simulink model "Motor_COM"  (R2024a)
settings: Solver=FixedStepAuto  StartTime=0.0  StopTime=10  FixedStep=MotorSampleTime/4  RelTol=1e-3
model workspace (MAT data in the model file):
  MotorSampleTime = 0.0025
libraries: instrumentseriallib x5, sldrtlib x1
settings Model: Creator=17739  LastModifiedBy=17739

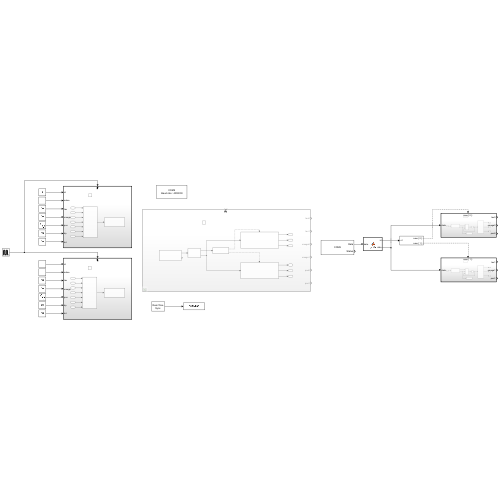
[thumbnail: Simulink's stored preview of the top-level diagram]
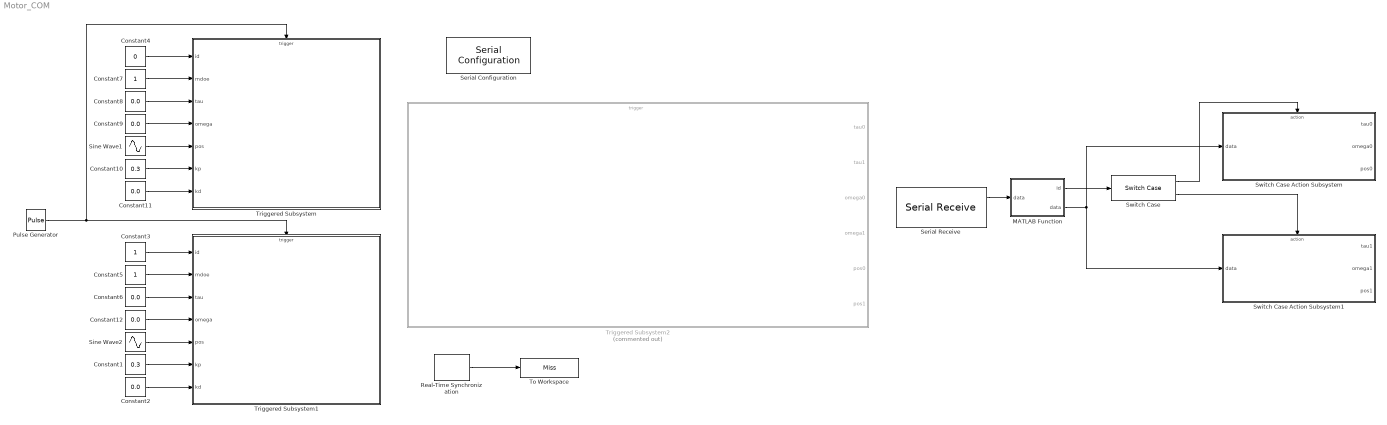
== system Motor_COM ==
  Constant1 : Constant  Value=0.3
  Constant10 : Constant  Value=0.3
  Constant{2,6,8..9,11..12} (6 alike) : Constant  Value=0.0
  Constant3 : Constant
  Constant4 : Constant  Value=0
  Constant5 : Constant
  Constant7 : Constant
  MATLAB Function : MATLAB Function  TreatAsAtomicUnit=on
  Pulse Generator : DiscretePulseGenerator  PulseType=Time based  Period=MotorSampleTime  PulseWidth=25
  Real-Time Synchronization : sldrtlib/Real-Time Synchronization  SampleTime=MotorSampleTime/4  MaxMissedTicks=inf  ShowMissedTicks=on  YieldWhenWaiting=off
  Serial Configuration : instrumentseriallib/Serial Configuration  Priority=-200000  PortSel=COM9  Port=COM9  ComPort=COM9  BaudRate=4000000  DataBits=8  Parity=none  StopBits=1  ByteOrder=little-endian  FlowControl=none  Timeout=0.02  SimulateUsing=Interpreted execution  BlockInModel=on  aMode=1
  Serial Receive : instrumentseriallib/Serial Receive  PortSel=COM9  Port=COM9  ComPort=COM9  DataType=uint8  SaveDataType=uint8  ToggleHeader=on  Header=[253 238]  ToggleDataSize=on  DataSize=14  ToggleTerminator=on  Terminator=<none>  CustomTerminator=[]  InputFormat=Row major  EnableBlockingMode=off  ActionDataUnavailable=Output last received value  ActionWhenDataUnavailable=Output last received value  CustomValue=0  SampleTime=MotorSampleTime/2  SimulateUsing=Interpreted execution  BlockInModel=on  aMode=1
  Sine Wave1 : Sin  Amplitude=pi  Frequency=pi/5  SampleTime=0
  Sine Wave2 : Sin  Amplitude=pi  Frequency=pi/5  SampleTime=0
  Switch Case : SwitchCase  CaseConditions={0,1}  ShowDefaultCase=off
  Switch Case Action Subsystem : Subsystem  TreatAsAtomicUnit=on
  Switch Case Action Subsystem1 : Subsystem  TreatAsAtomicUnit=on
  To Workspace : ToWorkspace  VariableName=Miss  SampleTime=-1
  Triggered Subsystem : Subsystem  TreatAsAtomicUnit=on
  Triggered Subsystem1 : Subsystem  TreatAsAtomicUnit=on
  Triggered Subsystem2 : Subsystem  Commented=on  TreatAsAtomicUnit=on
  wires:
  Real-Time Synchronization/1 -> To Workspace/1
  Switch Case/1 -> Switch Case Action Subsystem/Action
  Switch Case/2 -> Switch Case Action Subsystem1/Action
  MATLAB Function/2(data) -> Switch Case Action Subsystem1/1(data), Switch Case Action Subsystem/1(data)
  MATLAB Function/1(id) -> Switch Case/1
  Serial Receive/1 -> MATLAB Function/1("data ")
  Constant8/1 -> Triggered Subsystem/3(tau)
  Constant1/1 -> Triggered Subsystem1/6(kp)
  Constant6/1 -> Triggered Subsystem1/3(tau)
  Constant5/1 -> Triggered Subsystem1/2(mdoe)
  Constant9/1 -> Triggered Subsystem/4(omega)
  Constant10/1 -> Triggered Subsystem/6(kp)
  Constant4/1 -> Triggered Subsystem/1(id)
  Constant12/1 -> Triggered Subsystem1/4(omega)
  Pulse Generator/1 -> Triggered Subsystem/Trigger, Triggered Subsystem1/Trigger
  Constant11/1 -> Triggered Subsystem/7(kd)
  Constant3/1 -> Triggered Subsystem1/1(id)
  Constant2/1 -> Triggered Subsystem1/7(kd)
  Constant7/1 -> Triggered Subsystem/2(mdoe)
  Sine Wave2/1 -> Triggered Subsystem1/5(pos)
  Sine Wave1/1 -> Triggered Subsystem/5(pos)

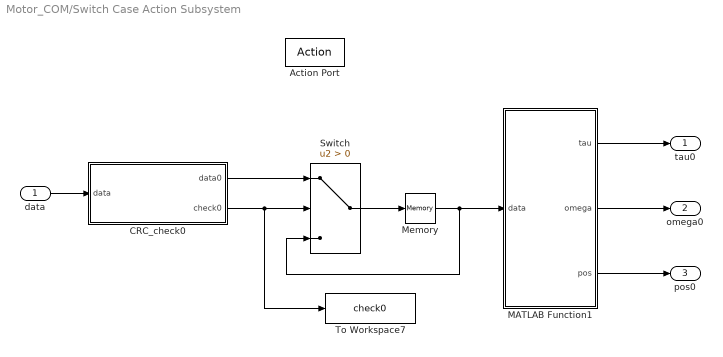
== system Motor_COM/Switch Case Action Subsystem ==
  data : Inport
  Action Port : ActionPort  ActionPortLabel=case [ 0 ]:
  CRC_check0 : MATLAB Function  TreatAsAtomicUnit=on
  MATLAB Function1 : MATLAB Function  TreatAsAtomicUnit=on
  Memory : Memory  InheritSampleTime=on
  Switch : Switch  Criteria=u2 > Threshold  SaturateOnIntegerOverflow=off  InputSameDT=off
  To Workspace7 : ToWorkspace  VariableName=check0  SampleTime=-1
  tau0 : Outport
  omega0 : Outport  Port=2
  pos0 : Outport  Port=3
  wires:
  CRC_check0/1(data0) -> Switch/1
  CRC_check0/2(check0) -> Switch/2, To Workspace7/1
  Memory/1 -> MATLAB Function1/1(data), Switch/3
  Switch/1 -> Memory/1
  data/1 -> CRC_check0/1(data)
  MATLAB Function1/1(tau) -> tau0/1
  MATLAB Function1/2(omega) -> omega0/1
  MATLAB Function1/3(pos) -> pos0/1

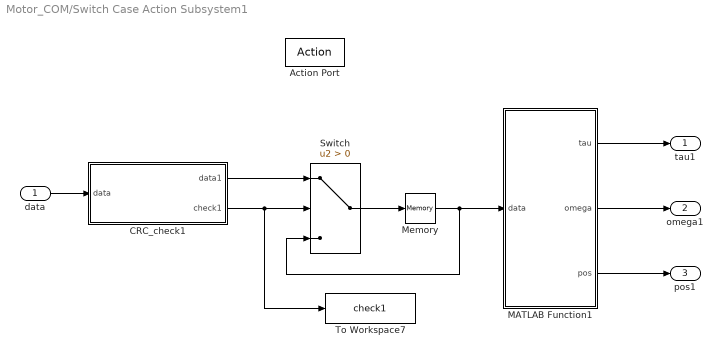
== system Motor_COM/Switch Case Action Subsystem1 ==
  data : Inport
  Action Port : ActionPort  ActionPortLabel=case [ 1 ]:
  CRC_check1 : MATLAB Function  TreatAsAtomicUnit=on
  MATLAB Function1 : MATLAB Function  TreatAsAtomicUnit=on
  Memory : Memory  InheritSampleTime=on
  Switch : Switch  Criteria=u2 > Threshold  SaturateOnIntegerOverflow=off  InputSameDT=off
  To Workspace7 : ToWorkspace  VariableName=check1  SampleTime=-1
  tau1 : Outport
  omega1 : Outport  Port=2
  pos1 : Outport  Port=3
  wires:
  CRC_check1/1(data1) -> Switch/1
  CRC_check1/2(check1) -> Switch/2, To Workspace7/1
  Memory/1 -> MATLAB Function1/1(data), Switch/3
  Switch/1 -> Memory/1
  data/1 -> CRC_check1/1(data)
  MATLAB Function1/1(tau) -> tau1/1
  MATLAB Function1/2(omega) -> omega1/1
  MATLAB Function1/3(pos) -> pos1/1

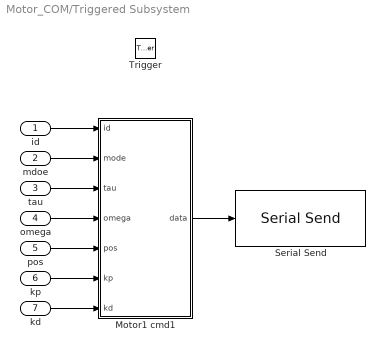
== system Motor_COM/Triggered Subsystem ==
  id : Inport
  mdoe : Inport  Port=2
  tau : Inport  Port=3
  omega : Inport  Port=4
  pos : Inport  Port=5
  kp : Inport  Port=6
  kd : Inport  Port=7
  Trigger : TriggerPort  VariantControl=(inherit)
  Motor1 cmd1 : MATLAB Function  TreatAsAtomicUnit=on
  Serial Send : instrumentseriallib/Serial Send  Priority=1  PortSel=COM9  Port=COM9  ComPort=COM9  Header=[]  Terminator=<none>  CustomTerminator=[]  EnableBlockingMode=off  SimulateUsing=Interpreted execution  BlockInModel=on  aMode=1
      settings: LibrarySourceBlock=c2000lib/Host Communication/Serial Send
  wires:
  tau/1 -> Motor1 cmd1/3(tau)
  mdoe/1 -> Motor1 cmd1/2(mode)
  kp/1 -> Motor1 cmd1/6(kp)
  id/1 -> Motor1 cmd1/1(id)
  omega/1 -> Motor1 cmd1/4(omega)
  kd/1 -> Motor1 cmd1/7(kd)
  pos/1 -> Motor1 cmd1/5(pos)
  Motor1 cmd1/1(data) -> Serial Send/1

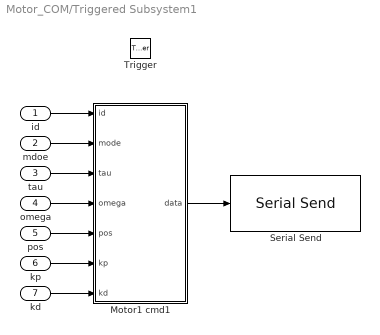
== system Motor_COM/Triggered Subsystem1 ==
  id : Inport
  mdoe : Inport  Port=2
  tau : Inport  Port=3
  omega : Inport  Port=4
  pos : Inport  Port=5
  kp : Inport  Port=6
  kd : Inport  Port=7
  Trigger : TriggerPort  TriggerType=falling  VariantControl=(inherit)
  Motor1 cmd1 : MATLAB Function  TreatAsAtomicUnit=on
  Serial Send : instrumentseriallib/Serial Send  Priority=1  PortSel=COM9  Port=COM9  ComPort=COM9  Header=[]  Terminator=<none>  CustomTerminator=[]  EnableBlockingMode=off  SimulateUsing=Interpreted execution  BlockInModel=on  aMode=1
      settings: LibrarySourceBlock=c2000lib/Host Communication/Serial Send
  wires:
  tau/1 -> Motor1 cmd1/3(tau)
  mdoe/1 -> Motor1 cmd1/2(mode)
  kp/1 -> Motor1 cmd1/6(kp)
  id/1 -> Motor1 cmd1/1(id)
  omega/1 -> Motor1 cmd1/4(omega)
  kd/1 -> Motor1 cmd1/7(kd)
  pos/1 -> Motor1 cmd1/5(pos)
  Motor1 cmd1/1(data) -> Serial Send/1

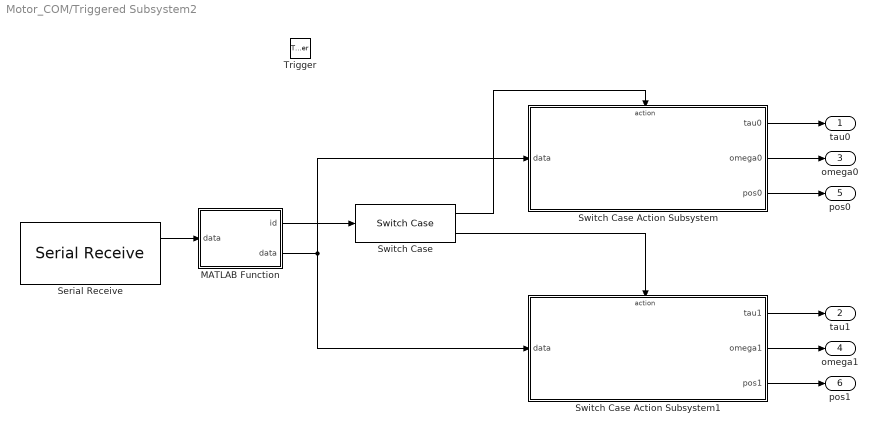
== system Motor_COM/Triggered Subsystem2 ==
  Trigger : TriggerPort  TriggerType=either  VariantControl=(inherit)
  MATLAB Function : MATLAB Function  TreatAsAtomicUnit=on
  Serial Receive : instrumentseriallib/Serial Receive  PortSel=COM9  Port=COM9  ComPort=COM9  DataType=uint8  SaveDataType=uint8  ToggleHeader=on  Header=[253 238]  ToggleDataSize=on  DataSize=14  ToggleTerminator=off  Terminator=<none>  CustomTerminator=[]  InputFormat=Row major  EnableBlockingMode=off  ActionDataUnavailable=Output last received value  ActionWhenDataUnavailable=Output last received value  CustomValue=0  SampleTime=-1  SimulateUsing=Interpreted execution  BlockInModel=on  aMode=1
  Switch Case : SwitchCase  CaseConditions={0,1}  ShowDefaultCase=off
  Switch Case Action Subsystem : Subsystem  TreatAsAtomicUnit=on
  Switch Case Action Subsystem1 : Subsystem  TreatAsAtomicUnit=on
  tau0 : Outport
  tau1 : Outport  Port=2
  omega0 : Outport  Port=3
  omega1 : Outport  Port=4
  pos0 : Outport  Port=5
  pos1 : Outport  Port=6
  wires:
  Serial Receive/1 -> MATLAB Function/1("data ")
  MATLAB Function/1(id) -> Switch Case/1
  MATLAB Function/2(data) -> Switch Case Action Subsystem1/1(data), Switch Case Action Subsystem/1(data)
  Switch Case/1 -> Switch Case Action Subsystem/Action
  Switch Case/2 -> Switch Case Action Subsystem1/Action
  Switch Case Action Subsystem/1(tau0) -> tau0/1
  Switch Case Action Subsystem1/1(tau1) -> tau1/1
  Switch Case Action Subsystem/2(omega0) -> omega0/1
  Switch Case Action Subsystem1/2(omega1) -> omega1/1
  Switch Case Action Subsystem/3(pos0) -> pos0/1
  Switch Case Action Subsystem1/3(pos1) -> pos1/1

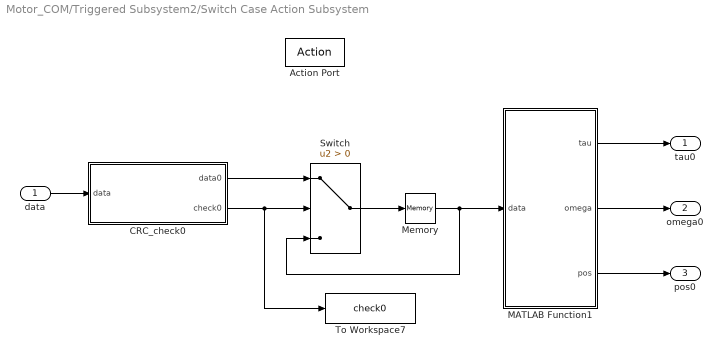
== system Motor_COM/Triggered Subsystem2/Switch Case Action Subsystem ==
  data : Inport
  Action Port : ActionPort  ActionPortLabel=case [ 0 ]:
  CRC_check0 : MATLAB Function  TreatAsAtomicUnit=on
  MATLAB Function1 : MATLAB Function  TreatAsAtomicUnit=on
  Memory : Memory  InheritSampleTime=on
  Switch : Switch  Criteria=u2 > Threshold  SaturateOnIntegerOverflow=off  InputSameDT=off
  To Workspace7 : ToWorkspace  VariableName=check0  SampleTime=-1
  tau0 : Outport
  omega0 : Outport  Port=2
  pos0 : Outport  Port=3
  wires:
  CRC_check0/1(data0) -> Switch/1
  CRC_check0/2(check0) -> Switch/2, To Workspace7/1
  Memory/1 -> MATLAB Function1/1(data), Switch/3
  Switch/1 -> Memory/1
  data/1 -> CRC_check0/1(data)
  MATLAB Function1/1(tau) -> tau0/1
  MATLAB Function1/2(omega) -> omega0/1
  MATLAB Function1/3(pos) -> pos0/1

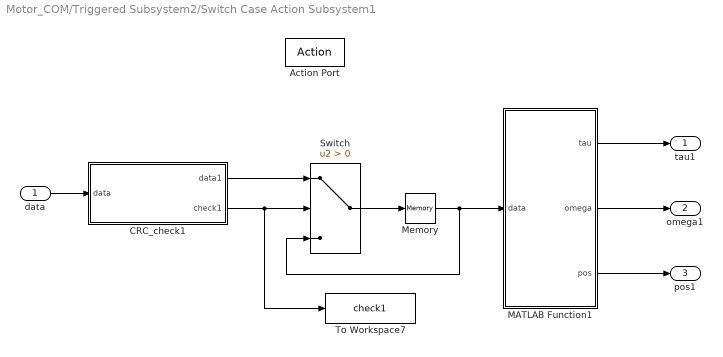
== system Motor_COM/Triggered Subsystem2/Switch Case Action Subsystem1 ==
  data : Inport
  Action Port : ActionPort  ActionPortLabel=case [ 1 ]:
  CRC_check1 : MATLAB Function  TreatAsAtomicUnit=on
  MATLAB Function1 : MATLAB Function  TreatAsAtomicUnit=on
  Memory : Memory  InheritSampleTime=on
  Switch : Switch  Criteria=u2 > Threshold  SaturateOnIntegerOverflow=off  InputSameDT=off
  To Workspace7 : ToWorkspace  VariableName=check1  SampleTime=-1
  tau1 : Outport
  omega1 : Outport  Port=2
  pos1 : Outport  Port=3
  wires:
  CRC_check1/1(data1) -> Switch/1
  CRC_check1/2(check1) -> Switch/2, To Workspace7/1
  Memory/1 -> MATLAB Function1/1(data), Switch/3
  Switch/1 -> Memory/1
  data/1 -> CRC_check1/1(data)
  MATLAB Function1/1(tau) -> tau1/1
  MATLAB Function1/2(omega) -> omega1/1
  MATLAB Function1/3(pos) -> pos1/1

== matlab function Motor_COM/Triggered Subsystem2/Switch Case Action Subsystem1/CRC_check1 ==
  data: data1 output; check1 output; data input
function [data1, check1] = CRC_Check1(data)
crc_ccitt_table = [
    0x0000, 0x1189, 0x2312, 0x329b, 0x4624, 0x57ad, 0x6536, 0x74bf, ...
    0x8c48, 0x9dc1, 0xaf5a, 0xbed3, 0xca6c, 0xdbe5, 0xe97e, 0xf8f7, ...
    0x1081, 0x0108, 0x3393, 0x221a, 0x56a5, 0x472c, 0x75b7, 0x643e, ...
    0x9cc9, 0x8d40, 0xbfdb, 0xae52, 0xdaed, 0xcb64, 0xf9ff, 0xe876, ...
    0x2102, 0x308b, 0x0210, 0x1399, 0x6726, 0x76af, 0x4434, 0x55bd, ...
    0xad4a, 0xbcc3, 0x8e58, 0x9fd1, 0xeb6e, 0xfae7, 0xc87c, 0xd9f5, ...
    0x3183, 0x200a, 0x1291, 0x0318, 0x77a7, 0x662e, 0x54b5, 0x453c, ...
    0xbdcb, 0xac42, 0x9ed9, 0x8f50, 0xfbef, 0xea66, 0xd8fd, 0xc974, ...
    0x4204, 0x538d, 0x6116, 0x709f, 0x0420, 0x15a9, 0x2732, 0x36bb, ...
    0xce4c, 0xdfc5, 0xed5e, 0xfcd7, 0x8868, 0x99e1, 0xab7a, 0xbaf3, ...
    0x5285, 0x430c, 0x7197, 0x601e, 0x14a1, 0x0528, 0x37b3, 0x263a, ...
    0xdecd, 0xcf44, 0xfddf, 0xec56, 0x98e9, 0x8960, 0xbbfb, 0xaa72, ...
    0x6306, 0x728f, 0x4014, 0x519d, 0x2522, 0x34ab, 0x0630, 0x17b9, ...
    0xef4e, 0xfec7, 0xcc5c, 0xddd5, 0xa96a, 0xb8e3, 0x8a78, 0x9bf1, ...
    0x7387, 0x620e, 0x5095, 0x411c, 0x35a3, 0x242a, 0x16b1, 0x0738, ...
    0xffcf, 0xee46, 0xdcdd, 0xcd54, 0xb9eb, 0xa862, 0x9af9, 0x8b70, ...
    0x8408, 0x9581, 0xa71a, 0xb693, 0xc22c, 0xd3a5, 0xe13e, 0xf0b7, ...
    0x0840, 0x19c9, 0x2b52, 0x3adb, 0x4e64, 0x5fed, 0x6d76, 0x7cff, ...
    0x9489, 0x8500, 0xb79b, 0xa612, 0xd2ad, 0xc324, 0xf1bf, 0xe036, ...
    0x18c1, 0x0948, 0x3bd3, 0x2a5a, 0x5ee5, 0x4f6c, 0x7df7, 0x6c7e, ...
    0xa50a, 0xb483, 0x8618, 0x9791, 0xe32e, 0xf2a7, 0xc03c, 0xd1b5, ...
    0x2942, 0x38cb, 0x0a50, 0x1bd9, 0x6f66, 0x7eef, 0x4c74, 0x5dfd, ...
    0xb58b, 0xa402, 0x9699, 0x8710, 0xf3af, 0xe226, 0xd0bd, 0xc134, ...
    0x39c3, 0x284a, 0x1ad1, 0x0b58, 0x7fe7, 0x6e6e, 0x5cf5, 0x4d7c, ...
    0xc60c, 0xd785, 0xe51e, 0xf497, 0x8028, 0x91a1, 0xa33a, 0xb2b3, ...
    0x4a44, 0x5bcd, 0x6956, 0x78df, 0x0c60, 0x1de9, 0x2f72, 0x3efb, ...
    0xd68d, 0xc704, 0xf59f, 0xe416, 0x90a9, 0x8120, 0xb3bb, 0xa232, ...
    0x5ac5, 0x4b4c, 0x79d7, 0x685e, 0x1ce1, 0x0d68, 0x3ff3, 0x2e7a, ...
    0xe70e, 0xf687, 0xc41c, 0xd595, 0xa12a, 0xb0a3, 0x8238, 0x93b1, ...
    0x6b46, 0x7acf, 0x4854, 0x59dd, 0x2d62, 0x3ceb, 0x0e70, 0x1ff9, ...
    0xf78f, 0xe606, 0xd49d, 0xc514, 0xb1ab, 0xa022, 0x92b9, 0x8330, ...
    0x7bc7, 0x6a4e, 0x58d5, 0x495c, 0x3de3, 0x2c6a, 0x1ef1, 0x0f78 ...
    ];

data1 = [253; 238; data];
crc = uint16(0);
for i = 1:14
    tableIndex = bitand(bitxor(crc, uint16(data1(i))), uint16(0xff));
    crc = bitxor(bitshift(crc, -8), crc_ccitt_table(tableIndex + 1));
end
check1 = false;
if typecast(uint8(data1(end-1:end)), 'uint16') == crc
    check1 = true;
end
end

== matlab function Motor_COM/Triggered Subsystem2/Switch Case Action Subsystem1/MATLAB Function1 ==
  data: data input size=[16 1]; tau output size=1; omega output size=1; pos output size=1
function [tau, omega, pos] = MotorData(data)
tau = double(typecast(uint8(data(4:5)), 'int16')) / 256;
omega = double(typecast(uint8(data(6:7)), 'int16')) / 256 * 2 * pi;
pos = double(typecast(uint8(data(8:11)), 'int32')) / 32768 * 2 * pi;
end

== matlab function Motor_COM/Triggered Subsystem/Motor1 cmd1 ==
  data: data output size=[1 17]; id input; mode input; tau input; omega input; pos input; kp input; kd input
function data = MotorCmd(id, mode, tau, omega, pos, kp, kd)
data = uint8([hex2dec('FE'), hex2dec('EE'), ...
    mode*16 + id, ...
    typecast(int16(fix(tau * 256)), 'uint8'), ...
    typecast(int16(fix(omega / (2 * pi) * 256)), 'uint8'), ...
    typecast(int32(fix(pos / (2 * pi) * 32768)), 'uint8'), ...
    typecast(int16(fix(kp * 1280)), 'uint8'), ...
    typecast(int16(fix(kd * 1280)), 'uint8'), ...
    0, 0]); % CRC16 计算稍后添加

% 计算并添加 CRC16 校验
crc = calculateCRC(data(1:end-2)); % 自定义 CRC 计算函数
data(end-1:end) = typecast(uint16(crc), 'uint8');
end

% 自定义 CRC 计算函数
function crc = calculateCRC(data)
crc_ccitt_table = [
    0x0000, 0x1189, 0x2312, 0x329b, 0x4624, 0x57ad, 0x6536, 0x74bf, ...
    0x8c48, 0x9dc1, 0xaf5a, 0xbed3, 0xca6c, 0xdbe5, 0xe97e, 0xf8f7, ...
    0x1081, 0x0108, 0x3393, 0x221a, 0x56a5, 0x472c, 0x75b7, 0x643e, ...
    0x9cc9, 0x8d40, 0xbfdb, 0xae52, 0xdaed, 0xcb64, 0xf9ff, 0xe876, ...
    0x2102, 0x308b, 0x0210, 0x1399, 0x6726, 0x76af, 0x4434, 0x55bd, ...
    0xad4a, 0xbcc3, 0x8e58, 0x9fd1, 0xeb6e, 0xfae7, 0xc87c, 0xd9f5, ...
    0x3183, 0x200a, 0x1291, 0x0318, 0x77a7, 0x662e, 0x54b5, 0x453c, ...
    0xbdcb, 0xac42, 0x9ed9, 0x8f50, 0xfbef, 0xea66, 0xd8fd, 0xc974, ...
    0x4204, 0x538d, 0x6116, 0x709f, 0x0420, 0x15a9, 0x2732, 0x36bb, ...
    0xce4c, 0xdfc5, 0xed5e, 0xfcd7, 0x8868, 0x99e1, 0xab7a, 0xbaf3, ...
    0x5285, 0x430c, 0x7197, 0x601e, 0x14a1, 0x0528, 0x37b3, 0x263a, ...
    0xdecd, 0xcf44, 0xfddf, 0xec56, 0x98e9, 0x8960, 0xbbfb, 0xaa72, ...
    0x6306, 0x728f, 0x4014, 0x519d, 0x2522, 0x34ab, 0x0630, 0x17b9, ...
    0xef4e, 0xfec7, 0xcc5c, 0xddd5, 0xa96a, 0xb8e3, 0x8a78, 0x9bf1, ...
    0x7387, 0x620e, 0x5095, 0x411c, 0x35a3, 0x242a, 0x16b1, 0x0738, ...
    0xffcf, 0xee46, 0xdcdd, 0xcd54, 0xb9eb, 0xa862, 0x9af9, 0x8b70, ...
    0x8408, 0x9581, 0xa71a, 0xb693, 0xc22c, 0xd3a5, 0xe13e, 0xf0b7, ...
    0x0840, 0x19c9, 0x2b52, 0x3adb, 0x4e64, 0x5fed, 0x6d76, 0x7cff, ...
    0x9489, 0x8500, 0xb79b, 0xa612, 0xd2ad, 0xc324, 0xf1bf, 0xe036, ...
    0x18c1, 0x0948, 0x3bd3, 0x2a5a, 0x5ee5, 0x4f6c, 0x7df7, 0x6c7e, ...
    0xa50a, 0xb483, 0x8618, 0x9791, 0xe32e, 0xf2a7, 0xc03c, 0xd1b5, ...
    0x2942, 0x38cb, 0x0a50, 0x1bd9, 0x6f66, 0x7eef, 0x4c74, 0x5dfd, ...
    0xb58b, 0xa402, 0x9699, 0x8710, 0xf3af, 0xe226, 0xd0bd, 0xc134, ...
    0x39c3, 0x284a, 0x1ad1, 0x0b58, 0x7fe7, 0x6e6e, 0x5cf5, 0x4d7c, ...
    0xc60c, 0xd785, 0xe51e, 0xf497, 0x8028, 0x91a1, 0xa33a, 0xb2b3, ...
    0x4a44, 0x5bcd, 0x6956, 0x78df, 0x0c60, 0x1de9, 0x2f72, 0x3efb, ...
    0xd68d, 0xc704, 0xf59f, 0xe416, 0x90a9, 0x8120, 0xb3bb, 0xa232, ...
    0x5ac5, 0x4b4c, 0x79d7, 0x685e, 0x1ce1, 0x0d68, 0x3ff3, 0x2e7a, ...
    0xe70e, 0xf687, 0xc41c, 0xd595, 0xa12a, 0xb0a3, 0x8238, 0x93b1, ...
    0x6b46, 0x7acf, 0x4854, 0x59dd, 0x2d62, 0x3ceb, 0x0e70, 0x1ff9, ...
    0xf78f, 0xe606, 0xd49d, 0xc514, 0xb1ab, 0xa022, 0x92b9, 0x8330, ...
    0x7bc7, 0x6a4e, 0x58d5, 0x495c, 0x3de3, 0x2c6a, 0x1ef1, 0x0f78 ...
    ];

crc = uint16(0);
for i = 1:length(data)
    tableIndex = bitand(bitxor(crc, uint16(data(i))), uint16(0xff));
    crc = bitxor(bitshift(crc, -8), crc_ccitt_table(tableIndex + 1));
end
end

== matlab function Motor_COM/MATLAB Function ==
  data: data input; id output; data output
function [id, data] = getID(data)
id = uint8(data(1)) - 16;
end

== matlab function Motor_COM/Triggered Subsystem1/Motor1 cmd1 ==
  data: data output size=[1 17]; id input; mode input; tau input; omega input; pos input; kp input; kd input
function data = MotorCmd(id, mode, tau, omega, pos, kp, kd)
data = uint8([hex2dec('FE'), hex2dec('EE'), ...
    mode*16 + id, ...
    typecast(int16(fix(tau * 256)), 'uint8'), ...
    typecast(int16(fix(omega / (2 * pi) * 256)), 'uint8'), ...
    typecast(int32(fix(pos / (2 * pi) * 32768)), 'uint8'), ...
    typecast(int16(fix(kp * 1280)), 'uint8'), ...
    typecast(int16(fix(kd * 1280)), 'uint8'), ...
    0, 0]); % CRC16 计算稍后添加

% 计算并添加 CRC16 校验
crc = calculateCRC(data(1:end-2)); % 自定义 CRC 计算函数
data(end-1:end) = typecast(uint16(crc), 'uint8');
pause(0.00125);
end

% 自定义 CRC 计算函数
function crc = calculateCRC(data)
crc_ccitt_table = [
    0x0000, 0x1189, 0x2312, 0x329b, 0x4624, 0x57ad, 0x6536, 0x74bf, ...
    0x8c48, 0x9dc1, 0xaf5a, 0xbed3, 0xca6c, 0xdbe5, 0xe97e, 0xf8f7, ...
    0x1081, 0x0108, 0x3393, 0x221a, 0x56a5, 0x472c, 0x75b7, 0x643e, ...
    0x9cc9, 0x8d40, 0xbfdb, 0xae52, 0xdaed, 0xcb64, 0xf9ff, 0xe876, ...
    0x2102, 0x308b, 0x0210, 0x1399, 0x6726, 0x76af, 0x4434, 0x55bd, ...
    0xad4a, 0xbcc3, 0x8e58, 0x9fd1, 0xeb6e, 0xfae7, 0xc87c, 0xd9f5, ...
    0x3183, 0x200a, 0x1291, 0x0318, 0x77a7, 0x662e, 0x54b5, 0x453c, ...
    0xbdcb, 0xac42, 0x9ed9, 0x8f50, 0xfbef, 0xea66, 0xd8fd, 0xc974, ...
    0x4204, 0x538d, 0x6116, 0x709f, 0x0420, 0x15a9, 0x2732, 0x36bb, ...
    0xce4c, 0xdfc5, 0xed5e, 0xfcd7, 0x8868, 0x99e1, 0xab7a, 0xbaf3, ...
    0x5285, 0x430c, 0x7197, 0x601e, 0x14a1, 0x0528, 0x37b3, 0x263a, ...
    0xdecd, 0xcf44, 0xfddf, 0xec56, 0x98e9, 0x8960, 0xbbfb, 0xaa72, ...
    0x6306, 0x728f, 0x4014, 0x519d, 0x2522, 0x34ab, 0x0630, 0x17b9, ...
    0xef4e, 0xfec7, 0xcc5c, 0xddd5, 0xa96a, 0xb8e3, 0x8a78, 0x9bf1, ...
    0x7387, 0x620e, 0x5095, 0x411c, 0x35a3, 0x242a, 0x16b1, 0x0738, ...
    0xffcf, 0xee46, 0xdcdd, 0xcd54, 0xb9eb, 0xa862, 0x9af9, 0x8b70, ...
    0x8408, 0x9581, 0xa71a, 0xb693, 0xc22c, 0xd3a5, 0xe13e, 0xf0b7, ...
    0x0840, 0x19c9, 0x2b52, 0x3adb, 0x4e64, 0x5fed, 0x6d76, 0x7cff, ...
    0x9489, 0x8500, 0xb79b, 0xa612, 0xd2ad, 0xc324, 0xf1bf, 0xe036, ...
    0x18c1, 0x0948, 0x3bd3, 0x2a5a, 0x5ee5, 0x4f6c, 0x7df7, 0x6c7e, ...
    0xa50a, 0xb483, 0x8618, 0x9791, 0xe32e, 0xf2a7, 0xc03c, 0xd1b5, ...
    0x2942, 0x38cb, 0x0a50, 0x1bd9, 0x6f66, 0x7eef, 0x4c74, 0x5dfd, ...
    0xb58b, 0xa402, 0x9699, 0x8710, 0xf3af, 0xe226, 0xd0bd, 0xc134, ...
    0x39c3, 0x284a, 0x1ad1, 0x0b58, 0x7fe7, 0x6e6e, 0x5cf5, 0x4d7c, ...
    0xc60c, 0xd785, 0xe51e, 0xf497, 0x8028, 0x91a1, 0xa33a, 0xb2b3, ...
    0x4a44, 0x5bcd, 0x6956, 0x78df, 0x0c60, 0x1de9, 0x2f72, 0x3efb, ...
    0xd68d, 0xc704, 0xf59f, 0xe416, 0x90a9, 0x8120, 0xb3bb, 0xa232, ...
    0x5ac5, 0x4b4c, 0x79d7, 0x685e, 0x1ce1, 0x0d68, 0x3ff3, 0x2e7a, ...
    0xe70e, 0xf687, 0xc41c, 0xd595, 0xa12a, 0xb0a3, 0x8238, 0x93b1, ...
    0x6b46, 0x7acf, 0x4854, 0x59dd, 0x2d62, 0x3ceb, 0x0e70, 0x1ff9, ...
    0xf78f, 0xe606, 0xd49d, 0xc514, 0xb1ab, 0xa022, 0x92b9, 0x8330, ...
    0x7bc7, 0x6a4e, 0x58d5, 0x495c, 0x3de3, 0x2c6a, 0x1ef1, 0x0f78 ...
    ];

crc = uint16(0);
for i = 1:length(data)
    tableIndex = bitand(bitxor(crc, uint16(data(i))), uint16(0xff));
    crc = bitxor(bitshift(crc, -8), crc_ccitt_table(tableIndex + 1));
end
end

== matlab function Motor_COM/Switch Case Action Subsystem/CRC_check0 ==
  data: data0 output; check0 output; data input
function [data0, check0] = CRC_Check0(data)
crc_ccitt_table = [
    0x0000, 0x1189, 0x2312, 0x329b, 0x4624, 0x57ad, 0x6536, 0x74bf, ...
    0x8c48, 0x9dc1, 0xaf5a, 0xbed3, 0xca6c, 0xdbe5, 0xe97e, 0xf8f7, ...
    0x1081, 0x0108, 0x3393, 0x221a, 0x56a5, 0x472c, 0x75b7, 0x643e, ...
    0x9cc9, 0x8d40, 0xbfdb, 0xae52, 0xdaed, 0xcb64, 0xf9ff, 0xe876, ...
    0x2102, 0x308b, 0x0210, 0x1399, 0x6726, 0x76af, 0x4434, 0x55bd, ...
    0xad4a, 0xbcc3, 0x8e58, 0x9fd1, 0xeb6e, 0xfae7, 0xc87c, 0xd9f5, ...
    0x3183, 0x200a, 0x1291, 0x0318, 0x77a7, 0x662e, 0x54b5, 0x453c, ...
    0xbdcb, 0xac42, 0x9ed9, 0x8f50, 0xfbef, 0xea66, 0xd8fd, 0xc974, ...
    0x4204, 0x538d, 0x6116, 0x709f, 0x0420, 0x15a9, 0x2732, 0x36bb, ...
    0xce4c, 0xdfc5, 0xed5e, 0xfcd7, 0x8868, 0x99e1, 0xab7a, 0xbaf3, ...
    0x5285, 0x430c, 0x7197, 0x601e, 0x14a1, 0x0528, 0x37b3, 0x263a, ...
    0xdecd, 0xcf44, 0xfddf, 0xec56, 0x98e9, 0x8960, 0xbbfb, 0xaa72, ...
    0x6306, 0x728f, 0x4014, 0x519d, 0x2522, 0x34ab, 0x0630, 0x17b9, ...
    0xef4e, 0xfec7, 0xcc5c, 0xddd5, 0xa96a, 0xb8e3, 0x8a78, 0x9bf1, ...
    0x7387, 0x620e, 0x5095, 0x411c, 0x35a3, 0x242a, 0x16b1, 0x0738, ...
    0xffcf, 0xee46, 0xdcdd, 0xcd54, 0xb9eb, 0xa862, 0x9af9, 0x8b70, ...
    0x8408, 0x9581, 0xa71a, 0xb693, 0xc22c, 0xd3a5, 0xe13e, 0xf0b7, ...
    0x0840, 0x19c9, 0x2b52, 0x3adb, 0x4e64, 0x5fed, 0x6d76, 0x7cff, ...
    0x9489, 0x8500, 0xb79b, 0xa612, 0xd2ad, 0xc324, 0xf1bf, 0xe036, ...
    0x18c1, 0x0948, 0x3bd3, 0x2a5a, 0x5ee5, 0x4f6c, 0x7df7, 0x6c7e, ...
    0xa50a, 0xb483, 0x8618, 0x9791, 0xe32e, 0xf2a7, 0xc03c, 0xd1b5, ...
    0x2942, 0x38cb, 0x0a50, 0x1bd9, 0x6f66, 0x7eef, 0x4c74, 0x5dfd, ...
    0xb58b, 0xa402, 0x9699, 0x8710, 0xf3af, 0xe226, 0xd0bd, 0xc134, ...
    0x39c3, 0x284a, 0x1ad1, 0x0b58, 0x7fe7, 0x6e6e, 0x5cf5, 0x4d7c, ...
    0xc60c, 0xd785, 0xe51e, 0xf497, 0x8028, 0x91a1, 0xa33a, 0xb2b3, ...
    0x4a44, 0x5bcd, 0x6956, 0x78df, 0x0c60, 0x1de9, 0x2f72, 0x3efb, ...
    0xd68d, 0xc704, 0xf59f, 0xe416, 0x90a9, 0x8120, 0xb3bb, 0xa232, ...
    0x5ac5, 0x4b4c, 0x79d7, 0x685e, 0x1ce1, 0x0d68, 0x3ff3, 0x2e7a, ...
    0xe70e, 0xf687, 0xc41c, 0xd595, 0xa12a, 0xb0a3, 0x8238, 0x93b1, ...
    0x6b46, 0x7acf, 0x4854, 0x59dd, 0x2d62, 0x3ceb, 0x0e70, 0x1ff9, ...
    0xf78f, 0xe606, 0xd49d, 0xc514, 0xb1ab, 0xa022, 0x92b9, 0x8330, ...
    0x7bc7, 0x6a4e, 0x58d5, 0x495c, 0x3de3, 0x2c6a, 0x1ef1, 0x0f78 ...
    ];

data0 = [253; 238; data];
crc = uint16(0);
for i = 1:14
    tableIndex = bitand(bitxor(crc, uint16(data0(i))), uint16(0xff));
    crc = bitxor(bitshift(crc, -8), crc_ccitt_table(tableIndex + 1));
end
check0 = false;
if typecast(uint8(data0(end-1:end)), 'uint16') == crc
    check0 = true;
end
end

== matlab function Motor_COM/Switch Case Action Subsystem/MATLAB Function1 ==
  data: data input size=[16 1]; tau output size=1; omega output size=1; pos output size=1
function [tau, omega, pos] = MotorData(data)
tau = double(typecast(uint8(data(4:5)), 'int16')) / 256;
omega = double(typecast(uint8(data(6:7)), 'int16')) / 256 * 2 * pi;
pos = double(typecast(uint8(data(8:11)), 'int32')) / 32768 * 2 * pi;
end

== matlab function Motor_COM/Switch Case Action Subsystem1/CRC_check1 ==
  data: data1 output; check1 output; data input
function [data1, check1] = CRC_Check1(data)
crc_ccitt_table = [
    0x0000, 0x1189, 0x2312, 0x329b, 0x4624, 0x57ad, 0x6536, 0x74bf, ...
    0x8c48, 0x9dc1, 0xaf5a, 0xbed3, 0xca6c, 0xdbe5, 0xe97e, 0xf8f7, ...
    0x1081, 0x0108, 0x3393, 0x221a, 0x56a5, 0x472c, 0x75b7, 0x643e, ...
    0x9cc9, 0x8d40, 0xbfdb, 0xae52, 0xdaed, 0xcb64, 0xf9ff, 0xe876, ...
    0x2102, 0x308b, 0x0210, 0x1399, 0x6726, 0x76af, 0x4434, 0x55bd, ...
    0xad4a, 0xbcc3, 0x8e58, 0x9fd1, 0xeb6e, 0xfae7, 0xc87c, 0xd9f5, ...
    0x3183, 0x200a, 0x1291, 0x0318, 0x77a7, 0x662e, 0x54b5, 0x453c, ...
    0xbdcb, 0xac42, 0x9ed9, 0x8f50, 0xfbef, 0xea66, 0xd8fd, 0xc974, ...
    0x4204, 0x538d, 0x6116, 0x709f, 0x0420, 0x15a9, 0x2732, 0x36bb, ...
    0xce4c, 0xdfc5, 0xed5e, 0xfcd7, 0x8868, 0x99e1, 0xab7a, 0xbaf3, ...
    0x5285, 0x430c, 0x7197, 0x601e, 0x14a1, 0x0528, 0x37b3, 0x263a, ...
    0xdecd, 0xcf44, 0xfddf, 0xec56, 0x98e9, 0x8960, 0xbbfb, 0xaa72, ...
    0x6306, 0x728f, 0x4014, 0x519d, 0x2522, 0x34ab, 0x0630, 0x17b9, ...
    0xef4e, 0xfec7, 0xcc5c, 0xddd5, 0xa96a, 0xb8e3, 0x8a78, 0x9bf1, ...
    0x7387, 0x620e, 0x5095, 0x411c, 0x35a3, 0x242a, 0x16b1, 0x0738, ...
    0xffcf, 0xee46, 0xdcdd, 0xcd54, 0xb9eb, 0xa862, 0x9af9, 0x8b70, ...
    0x8408, 0x9581, 0xa71a, 0xb693, 0xc22c, 0xd3a5, 0xe13e, 0xf0b7, ...
    0x0840, 0x19c9, 0x2b52, 0x3adb, 0x4e64, 0x5fed, 0x6d76, 0x7cff, ...
    0x9489, 0x8500, 0xb79b, 0xa612, 0xd2ad, 0xc324, 0xf1bf, 0xe036, ...
    0x18c1, 0x0948, 0x3bd3, 0x2a5a, 0x5ee5, 0x4f6c, 0x7df7, 0x6c7e, ...
    0xa50a, 0xb483, 0x8618, 0x9791, 0xe32e, 0xf2a7, 0xc03c, 0xd1b5, ...
    0x2942, 0x38cb, 0x0a50, 0x1bd9, 0x6f66, 0x7eef, 0x4c74, 0x5dfd, ...
    0xb58b, 0xa402, 0x9699, 0x8710, 0xf3af, 0xe226, 0xd0bd, 0xc134, ...
    0x39c3, 0x284a, 0x1ad1, 0x0b58, 0x7fe7, 0x6e6e, 0x5cf5, 0x4d7c, ...
    0xc60c, 0xd785, 0xe51e, 0xf497, 0x8028, 0x91a1, 0xa33a, 0xb2b3, ...
    0x4a44, 0x5bcd, 0x6956, 0x78df, 0x0c60, 0x1de9, 0x2f72, 0x3efb, ...
    0xd68d, 0xc704, 0xf59f, 0xe416, 0x90a9, 0x8120, 0xb3bb, 0xa232, ...
    0x5ac5, 0x4b4c, 0x79d7, 0x685e, 0x1ce1, 0x0d68, 0x3ff3, 0x2e7a, ...
    0xe70e, 0xf687, 0xc41c, 0xd595, 0xa12a, 0xb0a3, 0x8238, 0x93b1, ...
    0x6b46, 0x7acf, 0x4854, 0x59dd, 0x2d62, 0x3ceb, 0x0e70, 0x1ff9, ...
    0xf78f, 0xe606, 0xd49d, 0xc514, 0xb1ab, 0xa022, 0x92b9, 0x8330, ...
    0x7bc7, 0x6a4e, 0x58d5, 0x495c, 0x3de3, 0x2c6a, 0x1ef1, 0x0f78 ...
    ];

data1 = [253; 238; data];
crc = uint16(0);
for i = 1:14
    tableIndex = bitand(bitxor(crc, uint16(data1(i))), uint16(0xff));
    crc = bitxor(bitshift(crc, -8), crc_ccitt_table(tableIndex + 1));
end
check1 = false;
if typecast(uint8(data1(end-1:end)), 'uint16') == crc
    check1 = true;
end
end

== matlab function Motor_COM/Switch Case Action Subsystem1/MATLAB Function1 ==
  data: data input size=[16 1]; tau output size=1; omega output size=1; pos output size=1
function [tau, omega, pos] = MotorData(data)
tau = double(typecast(uint8(data(4:5)), 'int16')) / 256;
omega = double(typecast(uint8(data(6:7)), 'int16')) / 256 * 2 * pi;
pos = double(typecast(uint8(data(8:11)), 'int32')) / 32768 * 2 * pi;
end

== matlab function Motor_COM/Triggered Subsystem2/MATLAB Function ==
  data: data input; id output; data output
function [id, data] = getID(data)
id = uint8(data(1)) - 16;
end

== matlab function Motor_COM/Triggered Subsystem2/Switch Case Action Subsystem/CRC_check0 ==
  data: data0 output; check0 output; data input
function [data0, check0] = CRC_Check0(data)
crc_ccitt_table = [
    0x0000, 0x1189, 0x2312, 0x329b, 0x4624, 0x57ad, 0x6536, 0x74bf, ...
    0x8c48, 0x9dc1, 0xaf5a, 0xbed3, 0xca6c, 0xdbe5, 0xe97e, 0xf8f7, ...
    0x1081, 0x0108, 0x3393, 0x221a, 0x56a5, 0x472c, 0x75b7, 0x643e, ...
    0x9cc9, 0x8d40, 0xbfdb, 0xae52, 0xdaed, 0xcb64, 0xf9ff, 0xe876, ...
    0x2102, 0x308b, 0x0210, 0x1399, 0x6726, 0x76af, 0x4434, 0x55bd, ...
    0xad4a, 0xbcc3, 0x8e58, 0x9fd1, 0xeb6e, 0xfae7, 0xc87c, 0xd9f5, ...
    0x3183, 0x200a, 0x1291, 0x0318, 0x77a7, 0x662e, 0x54b5, 0x453c, ...
    0xbdcb, 0xac42, 0x9ed9, 0x8f50, 0xfbef, 0xea66, 0xd8fd, 0xc974, ...
    0x4204, 0x538d, 0x6116, 0x709f, 0x0420, 0x15a9, 0x2732, 0x36bb, ...
    0xce4c, 0xdfc5, 0xed5e, 0xfcd7, 0x8868, 0x99e1, 0xab7a, 0xbaf3, ...
    0x5285, 0x430c, 0x7197, 0x601e, 0x14a1, 0x0528, 0x37b3, 0x263a, ...
    0xdecd, 0xcf44, 0xfddf, 0xec56, 0x98e9, 0x8960, 0xbbfb, 0xaa72, ...
    0x6306, 0x728f, 0x4014, 0x519d, 0x2522, 0x34ab, 0x0630, 0x17b9, ...
    0xef4e, 0xfec7, 0xcc5c, 0xddd5, 0xa96a, 0xb8e3, 0x8a78, 0x9bf1, ...
    0x7387, 0x620e, 0x5095, 0x411c, 0x35a3, 0x242a, 0x16b1, 0x0738, ...
    0xffcf, 0xee46, 0xdcdd, 0xcd54, 0xb9eb, 0xa862, 0x9af9, 0x8b70, ...
    0x8408, 0x9581, 0xa71a, 0xb693, 0xc22c, 0xd3a5, 0xe13e, 0xf0b7, ...
    0x0840, 0x19c9, 0x2b52, 0x3adb, 0x4e64, 0x5fed, 0x6d76, 0x7cff, ...
    0x9489, 0x8500, 0xb79b, 0xa612, 0xd2ad, 0xc324, 0xf1bf, 0xe036, ...
    0x18c1, 0x0948, 0x3bd3, 0x2a5a, 0x5ee5, 0x4f6c, 0x7df7, 0x6c7e, ...
    0xa50a, 0xb483, 0x8618, 0x9791, 0xe32e, 0xf2a7, 0xc03c, 0xd1b5, ...
    0x2942, 0x38cb, 0x0a50, 0x1bd9, 0x6f66, 0x7eef, 0x4c74, 0x5dfd, ...
    0xb58b, 0xa402, 0x9699, 0x8710, 0xf3af, 0xe226, 0xd0bd, 0xc134, ...
    0x39c3, 0x284a, 0x1ad1, 0x0b58, 0x7fe7, 0x6e6e, 0x5cf5, 0x4d7c, ...
    0xc60c, 0xd785, 0xe51e, 0xf497, 0x8028, 0x91a1, 0xa33a, 0xb2b3, ...
    0x4a44, 0x5bcd, 0x6956, 0x78df, 0x0c60, 0x1de9, 0x2f72, 0x3efb, ...
    0xd68d, 0xc704, 0xf59f, 0xe416, 0x90a9, 0x8120, 0xb3bb, 0xa232, ...
    0x5ac5, 0x4b4c, 0x79d7, 0x685e, 0x1ce1, 0x0d68, 0x3ff3, 0x2e7a, ...
    0xe70e, 0xf687, 0xc41c, 0xd595, 0xa12a, 0xb0a3, 0x8238, 0x93b1, ...
    0x6b46, 0x7acf, 0x4854, 0x59dd, 0x2d62, 0x3ceb, 0x0e70, 0x1ff9, ...
    0xf78f, 0xe606, 0xd49d, 0xc514, 0xb1ab, 0xa022, 0x92b9, 0x8330, ...
    0x7bc7, 0x6a4e, 0x58d5, 0x495c, 0x3de3, 0x2c6a, 0x1ef1, 0x0f78 ...
    ];

data0 = [253; 238; data];
crc = uint16(0);
for i = 1:14
    tableIndex = bitand(bitxor(crc, uint16(data0(i))), uint16(0xff));
    crc = bitxor(bitshift(crc, -8), crc_ccitt_table(tableIndex + 1));
end
check0 = false;
if typecast(uint8(data0(end-1:end)), 'uint16') == crc
    check0 = true;
end
end

== matlab function Motor_COM/Triggered Subsystem2/Switch Case Action Subsystem/MATLAB Function1 ==
  data: data input size=[16 1]; tau output size=1; omega output size=1; pos output size=1
function [tau, omega, pos] = MotorData(data)
tau = double(typecast(uint8(data(4:5)), 'int16')) / 256;
omega = double(typecast(uint8(data(6:7)), 'int16')) / 256 * 2 * pi;
pos = double(typecast(uint8(data(8:11)), 'int32')) / 32768 * 2 * pi;
end
